simulink model "stage3"  (Simulink 7.7)
settings: Solver=ode45  StartTime=0.0  StopTime=20  RelTol=1e-3
libraries: powerlib x4, simulink x2
settings Model: Creator=Vikas  LastModifiedBy=HASANTH

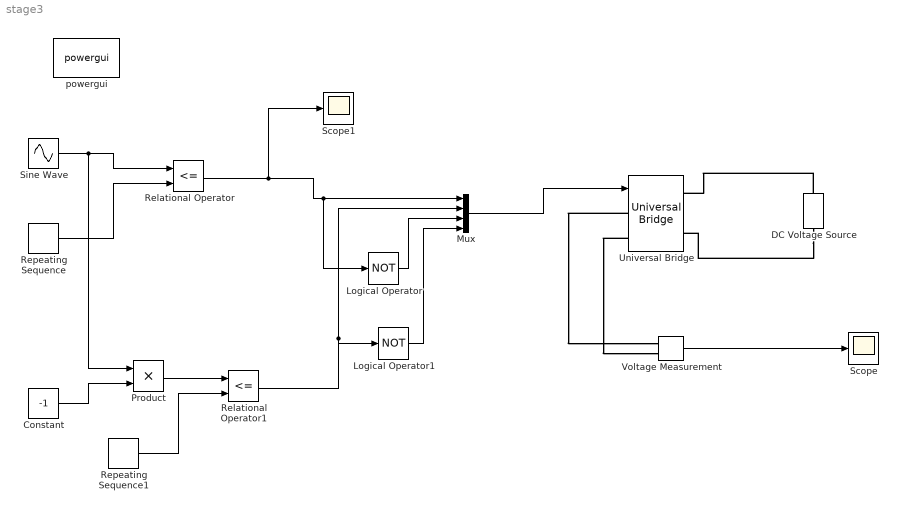
== system stage3 ==
  Constant : Constant  Value=-1
  DC Voltage Source : powerlib/Electrical Sources/DC Voltage Source  SystemSampleTime=-1  Amplitude=15  Measurements=None
  Logical Operator : Logic  Operator=NOT  AllPortsSameDT=off  OutDataTypeStr=boolean
  Logical Operator1 : Logic  Operator=NOT  AllPortsSameDT=off  OutDataTypeStr=boolean
  Mux : Mux
  Product : Product  RndMeth=Zero
  Relational Operator : RelationalOperator  Operator=<=  OutDataTypeStr=boolean
  Relational Operator1 : RelationalOperator  Operator=<=  OutDataTypeStr=boolean
  Repeating Sequence : simulink/Sources/Repeating Sequence  SystemSampleTime=-1  rep_seq_t=[0 0.5/1200 1/1200]  rep_seq_y=[-1 1 -1]
  Repeating Sequence1 : simulink/Sources/Repeating Sequence  SystemSampleTime=-1  rep_seq_t=[0 0.5/1200 1/1200]  rep_seq_y=[-1 1 -1]
  Scope : Scope
      settings: YMin=-50  YMax=50
  Scope1 : Scope
      settings: YMin=0  YMax=20
  Sine Wave : Sin  Amplitude=10  Frequency=300  SampleTime=0
  Universal Bridge : powerlib/Power Electronics/Universal Bridge  SystemSampleTime=-1  Arms=2  SnubberResistance=1e5  SnubberCapacitance=inf  Device=MOSFET / Diodes  Ron=1e-3  Lon=0  ForwardVoltages="[  0  0  ]"  ForwardVoltage=0  GTOparameters=[ 10e-6 , 20e-6 ]  IGBTparameters=[ 1e-6 , 2e-6 ]  Measurements=None  Measurements_2=None  converterType=Rectifier
  Voltage Measurement : powerlib/Measurements/Voltage Measurement  SystemSampleTime=-1  PhasorSimulation=off  OutputType=Complex  PSBequivalent=0
  powergui : powerlib/powergui  Priority=1  SystemSampleTime=-1  SimulationMode=Continuous  SampleTime=50e-6  frequency=60  SPID=off  DisableSnubberDevices=off  DisableRonSwitches=off  DisableVfSwitches=off  SwTol=0  Interpol=off  DisplayEquations=off  FunctionMessages=off  frequencyindice=0  Pbase=100e6  ErrMax=1e-4  Iterations=50  UnitsV=kV  UnitsW=MW  echomessages=off  HookPort=off  EnableUseOfTLC=off  x0status=blocks  RestoreLinks=warning  ResistiveCurrentMeasurement=off  Ylog=off  Xlog=on  ShowGrid=off  save=off  variable=ZData  ZoomFFT=off  StartTime=0.0  cycles=1  DisplayStyle=1  FreqAxis=off  MaxFrequency=1000  frequencyindicesteady=1  display=off  methode=off
  wires:
  Sine Wave/1 -> Relational Operator/1, Product/1
  Repeating Sequence/1 -> Relational Operator/2
  Relational Operator/1 -> Mux/1, Logical Operator/1, Scope1/1
  Constant/1 -> Product/2
  Product/1 -> Relational Operator1/1
  Repeating Sequence1/1 -> Relational Operator1/2
  Relational Operator1/1 -> Mux/2, Logical Operator1/1
  Logical Operator/1 -> Mux/3
  Logical Operator1/1 -> Mux/4
  Mux/1 -> Universal Bridge/1
  Voltage Measurement/1 -> Scope/1
  connections:
  DC Voltage Source/RConn1 -- Universal Bridge/RConn1
  DC Voltage Source/LConn1 -- Universal Bridge/RConn2
  Universal Bridge/LConn2 -- Voltage Measurement/LConn2
  Universal Bridge/LConn1 -- Voltage Measurement/LConn1
